simulink model "SimpleFMU"  (R2024b)
settings: Solver=VariableStepAuto  StartTime=0.0  StopTime=10.0  RelTol=1e-3
settings Model: Creator=mails  LastModifiedBy=mails

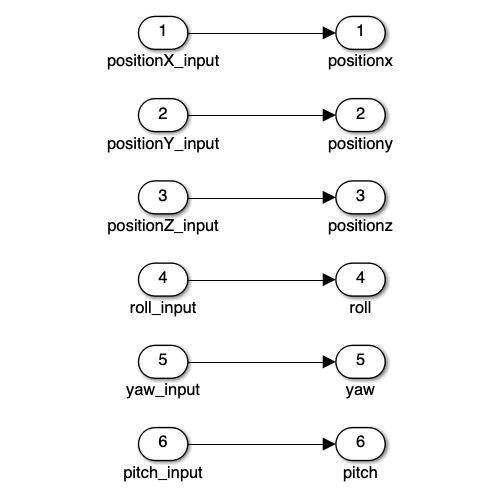
[thumbnail: Simulink's stored preview of the top-level diagram]
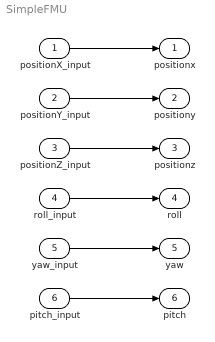
== system SimpleFMU ==
  positionX_input : Inport
  positionY_input : Inport  Port=2
  positionZ_input : Inport  Port=3
  roll_input : Inport  Port=4
  yaw_input : Inport  Port=5
  pitch_input : Inport  Port=6
  positionx : Outport
  positiony : Outport  Port=2
  positionz : Outport  Port=3
  roll : Outport  Port=4
  yaw : Outport  Port=5
  pitch : Outport  Port=6
  wires:
  positionX_input/1 -> positionx/1
  positionY_input/1 -> positiony/1
  positionZ_input/1 -> positionz/1
  roll_input/1 -> roll/1
  yaw_input/1 -> yaw/1
  pitch_input/1 -> pitch/1
